simulink model "main_sim_adapt_Gref_SP"  (Simulink 7.2)
settings: Solver=ode2  SolverMode=SingleTasking  StartTime=0.0  StopTime=tsim_max  FixedStep=dtsim  RelTol=1e-3
StopFcn:
  | %mkplt
values from neighbouring files (symbols this model uses):
  aero_surf_qbar_off = get_value('aero_surf_qbar_off')    [setup_claw.m]
  aero_surf_qbar_on = get_value('aero_surf_qbar_on')    [setup_claw.m]
  assertion_time = get_value('assertion_time')    [setup_sim.m]
  att_cmd_select = get_value('att_cmd_select')    [setup_sim.m]
  att_trim_IC = orientation.att'    [setup_claw.m]
  att_type_numbers = cell2mat(struct2cell(att_type))    [setup_constants.m]
  chi_trim_IC = orientation.Vchigam(2)    [setup_claw.m]
  command_time = engage_time + 2.0    [setup_sim.m]
  compute_all_rate_cols = get_value('compute_all_rate_cols')    [setup_claw.m]
  compute_all_vel_cols = get_value('compute_all_vel_cols')    [setup_claw.m]
  da_trim_IC = tmp(1)    [setup_claw.m]
  dc_L2W_IC = orientation.dc_L2W    [setup_claw.m]
  de_trim_IC = tmp(2)    [setup_claw.m]
  dr_trim_IC = tmp(3)    [setup_claw.m]
  dtsim = get_value('dtsim')    [setup_sim.m]
  E_trim_IC = MACH_pos_IC(2)    [setup_claw.m]
  Ed_trim_IC = MACH_vel_IC(2)    [setup_claw.m]
  gain_set = gain_set_next    (= 1)    [setup_claw.m]
  gain_var_struct = rmfield(gain_var_struct,setdiff(fieldnames(gain_var_struct),{'name','size'}))    [setup_claw.m]
  gamma_trim_IC = orientation.Vchigam(3)    [setup_claw.m]
  h_trim_IC = MACH_pos_IC(3)    [setup_claw.m]
  hd_trim_IC = MACH_vel_IC(3)    [setup_claw.m]
  ideal_vel_Kb = MACH_vel_Kb(1)    [setup_sim.m]
  MACH = rmfield(MACH,'vel_throt_lrlim')    [setup_claw.m]
  MACH_att_fb = get_value('MACH_att_fb','onerror',0)    [setup_claw.m]
  MACH_att_int_IC = (1-MACH_att_Kc).*MACH_quat_IC'    [setup_ideal.m]
  MACH_att_Kb = repval(att_kbnom,MACH.att_num_cv)    [setup_claw.m]
  MACH_att_Kc = Ki2Kc(MACH_att_Ki)    [setup_ideal.m]
  MACH_att_Ki = repval(att_fi,MACH.att_num_cv)    [setup_claw.m]
  MACH_gain_mat = vertcat(MACH_gain_mat, this_gain_mat)    [setup_claw.m]
  MACH_mass_IC = obac_params.mass_IC    [setup_claw.m]
  MACH_pos_IC = x_obac_IC(MACH.NEh_idx)    [setup_claw.m]
  MACH_pos_int_IC = (1-MACH_pos_Kc).*MACH_pos_IC' + MACH_vel_IC'./MACH_pos_Kb    [setup_ideal.m]
  MACH_pos_Kb = repval(pos_kbnom,MACH.pos_num_cv)    [setup_claw.m]
  MACH_pos_Kc = Ki2Kc(MACH_pos_Ki)    [setup_ideal.m]
  MACH_pos_Ki = repval(pos_fi,MACH.pos_num_cv)    [setup_claw.m]
  MACH_pqr_Bmat_IC = Bo(MACH.pqr_idx,MACH.pqr_u_idx)    [setup_claw.m]
  MACH_pqr_IC = pqr_trim_IC    [setup_claw.m]
  MACH_pqr_int_IC = (1-MACH_pqr_Kc).*MACH_pqr_IC'    [setup_ideal.m]
  MACH_pqr_Kb = repval(pqr_kbnom,MACH.pqr_num_cv)    [setup_claw.m]
  MACH_pqr_Kc = Ki2Kc(MACH_pqr_Ki)    [setup_ideal.m]
  MACH_pqr_Ki = repval(pqr_fi,MACH.pqr_num_cv)    [setup_claw.m]
  MACH_pqr_u_IC = [ vanes_trim_IC; tvc_trim_IC; rcs_trim_IC ]    [setup_claw.m]
  MACH_quat_IC = quat_trim_IC    [setup_claw.m]
  MACH_throttle_IC = throttle_trim_IC    [setup_claw.m]
  MACH_U_nom_IC = zeros(MACH.num_u,1)    [setup_claw.m]
  MACH_vel_Bmat_IC = MACH_vel_Bmat_IC*inv(vel_perts)    [setup_claw.m]
  MACH_vel_cvdnom_IC = repval(get_value('vel_cvdnom_IC','onerror',MACH_vel_cvdnom_IC),length(MACH_vel_cvdnom_IC))'    [setup_claw.m]
  MACH_vel_IC = orientation.NdEdhd'    [setup_claw.m]
  MACH_vel_int_IC = (1-MACH_vel_Kc).*MACH_vel_IC'    [setup_ideal.m]
  MACH_vel_Kb = repval(vel_kbnom,MACH.vel_num_cv)    [setup_claw.m]
  MACH_vel_Kc = Ki2Kc(MACH_vel_Ki)    [setup_ideal.m]
  MACH_vel_Ki = repval(vel_fi,MACH.vel_num_cv)    [setup_claw.m]
  MACH_vel_uold_IC = [ MACH_quat_IC; MACH_throttle_IC ]    [setup_claw.m]
  N_trim_IC = MACH_pos_IC(1)    [setup_claw.m]
  Nd_trim_IC = MACH_vel_IC(1)    [setup_claw.m]
  obac_params = define_model('obac', get_value('obac_model_type'))    [setup_claw.m]
  pos_cmd_select = get_value('pos_cmd_select')    [setup_sim.m]
  pqr_trim_IC = [ 0 0 0 ]'    [setup_claw.m]
  rate_cmd_select = get_value('rate_cmd_select')    [setup_sim.m]
  rcs_cvddes_thresh = get_value('rcs_cvddes_thresh')    [setup_claw.m]
  reset_camcmd_on_entry = get_value('reset_camcmd_on_entry')    [setup_claw.m]
  throttle_trim_IC = u_obac_IC(MACH.throttle_idx)    [setup_claw.m]
  trac_params = define_model('trac', get_value('trac_model_type','onerror',obac_params.model_type))    [setup_sim.m]
  use_auto_att_type = get_value('use_auto_att_type','onerror',0)    [setup_claw.m]
  use_eow_as_iv = get_value('use_eow_as_iv')    [setup_claw.m]
  use_full_surf_cmd = get_value('use_full_surf_cmd')    [setup_sim.m]
  use_nav = get_value('use_nav')    [setup_claw.m]
  use_NdEdh_pos = get_value('use_NdEdh_pos')    [setup_claw.m]
  use_pos_fltpath_lim = get_value('use_pos_fltpath_lim')    [setup_claw.m]
  use_throt_estimate = get_value('use_throt_estimate')    [setup_claw.m]
  use_variable_mass = get_value('use_variable_mass')    [setup_claw.m]
  use_wind_est = get_value('use_wind_est')    [setup_claw.m]
  V_trim_IC = orientation.Vchigam(1)    [setup_claw.m]
  vel_cmd_ramp_time = get_value('vel_cmd_ramp_time')    [setup_claw.m]
  vel_cmd_select = get_value('vel_cmd_select')    [setup_sim.m]
  x_trac_IC = x_obac_IC    [setup_sim.m]
undefined symbols (not defined in the file or in its folder): accel_cmd, alpha_trim, Am, att_type, B1, bb_ellipsoid, bb_params, Bm, C, constants, cosA, DiscIntNeverNeededParam, DZkx, DZtheta, E_rwy, Ed_cmd, eow_boundary, flag_autoadapt, flag_exsig, flag_uad, full_surf_llim, full_surf_ulim, gam_cmd_descent, gam_cmd_preflare, gamdot_cmd_descent, gamdot_cmd_flare, gamdot_cmd_preflare, Gamtheta, Gamx, hd_cmd, in_error_thresh, in_exsig_vecin, in_exsig_vecout, in_reset_stoptime, in_t_exsig, in_t_timer, in_tadaptoff_forced, in_tadapton_forced, Kb, Kxhat0, Kxnom, Kxstar, max_chi_cmd, max_LOS_rate, max_vel_cmd, min_chi_cmd, min_vel_cmd, modes, N_rwy, Nd_cmd, Nrbf, P, pos, Sig, sinA, target_pos_IC, target_range_blind, target_range_detect, target_range_homing, target_vel_IC ... (+11)
libraries: simulink x44, utility_lib x36, mach_lib x24, model_lib x13, simulink_need_slupdate x8, models x8
(part 5 of 8)

== system main_sim_adapt_Gref_SP/claw_main/input processing/mode dependent stick processing/rampin vel_cmd ==
  mode : Inport  OutDataType=sfix(16)  OutScaling=2^0
  command_in : Inport  Port=2  OutDataType=sfix(16)  OutScaling=2^0
  NEh_dot : Inport  Port=3  OutDataType=sfix(16)  OutScaling=2^0
  Compare To Constant : simulink/Logic and Bit Operations/Compare To Constant  SystemSampleTime=-1  relop=<=  const=modes.att  LogicOutDataTypeMode=boolean  ZeroCross=off
  Compare To Constant1 : simulink/Logic and Bit Operations/Compare To Constant  SystemSampleTime=-1  relop===  const=modes.vel  LogicOutDataTypeMode=boolean  ZeroCross=off
  Constant : Constant  Value=MACH.dt/max(vel_cmd_ramp_time,MACH.dt)  OutDataType=sfix(16)  OutScaling=2^0
  Constant1 : Constant  OutDataType=sfix(16)  OutScaling=2^0
  Constant2 : Constant  Value=0  OutDataType=sfix(16)  OutScaling=2^0
  Logical Operator : Logic  AllPortsSameDT=off
  MinMax : MinMax  Function=max  Inputs=2  OutDataType=sfix(16)  OutScaling=2^0
  Product : Product  OutDataType=sfix(16)  OutScaling=2^0  RndMeth=Zero
  Product1 : Product  OutDataType=sfix(16)  OutScaling=2^0  RndMeth=Zero
  Sum : Sum  Inputs=-+|  OutDataType=sfix(16)  OutScaling=2^0
  Sum2 : Sum  Inputs=|++  OutDataType=sfix(16)  OutScaling=2^0
  Sum3 : Sum  Inputs=|+-  OutDataType=sfix(16)  OutScaling=2^0
  Switch : Switch  Threshold=0.5
  Switch1 : Switch  Threshold=0.5
  Unit Delay : UnitDelay  Orientation=left  SampleTime=-1
  Unit Delay1 : UnitDelay  SampleTime=-1
  Unit Delay2 : UnitDelay  Orientation=left  SampleTime=-1
  set vel cmd : Assignment  IndexOptions=Index vector (dialog)  Indices=[1 2 4]  OutputSizes=[1 1]
  vel cmd : Selector  InputPortWidth=4  IndexOptions=Index vector (dialog)  Indices=[1 2 4]  OutputSizes=1
  command_out : Outport  OutDataType=sfix(16)  OutScaling=2^0
  wires:
  Unit Delay2/1 -> Product1/2
  Logical Operator/1 -> Switch/2, Switch1/2
  Compare To Constant1/1 -> Logical Operator/2, Product1/1
  Compare To Constant/1 -> Logical Operator/1
  Unit Delay1/1 -> Compare To Constant/1
  mode/1 -> Unit Delay1/1, Compare To Constant1/1
  Unit Delay/1 -> Switch/3
  Switch/1 -> Unit Delay/1, Product/1
  NEh_dot/1 -> Sum/2
  Sum/1 -> Switch/1
  set vel cmd/1 -> command_out/1
  vel cmd/1 -> Sum2/1, Sum/1
  command_in/1 -> set vel cmd/1, vel cmd/1
  Sum2/1 -> set vel cmd/2
  Product1/1 -> Switch1/3
  Constant1/1 -> Switch1/1
  Switch1/1 -> Sum3/1
  Product/1 -> Sum2/2
  Sum3/1 -> MinMax/2
  Constant/1 -> Sum3/2
  MinMax/1 -> Product/2, Unit Delay2/1
  Constant2/1 -> MinMax/1

== system main_sim_adapt_Gref_SP/claw_main/input processing/mode dependent stick processing/set command selection switches ==
  accel_cmd_sw : Inport  OutDataType=sfix(16)  OutScaling=2^0
  CLAW_mode : Inport  Port=2  OutDataType=sfix(16)  OutScaling=2^0
  Bus Creator : BusCreator
  Constant : Constant  Value=MACH.select_cmd_array  OutDataType=sfix(16)  OutScaling=2^0
  Demux : Demux  Outputs=[4 5 4 4]
  Reshape : Reshape
  Selector : Selector  NumberOfDimensions=2  IndexMode=Zero-based  InputPortWidth=3  IndexOptions=Select all,Index vector (port)  Indices=-1,1  OutputSizes=1
  modify for accel cmd submode : Subsystem
  select_cmd : Outport  OutDataType=sfix(16)  OutScaling=2^0
  wires:
  Constant/1 -> Selector/1
  CLAW_mode/1 -> Selector/2
  Selector/1 -> Reshape/1
  Demux/1 -> Bus Creator/1  "rate"
  Demux/2 -> Bus Creator/2  "att"
  Demux/3 -> Bus Creator/3  "vel"
  Demux/4 -> Bus Creator/4  "pos"
  Reshape/1 -> Demux/1
  modify for accel cmd submode/1(select_cmd) -> select_cmd/1
  Bus Creator/1 -> modify for accel cmd submode/1(select_cmd_in)
  accel_cmd_sw/1 -> modify for accel cmd submode/2(accel_cmd_sw)

== system main_sim_adapt_Gref_SP/claw_main/input processing/mode dependent stick processing/table iv computation ==
  x_est : Inport  OutDataType=sfix(16)  OutScaling=2^0
  Bus Creator : BusCreator  Inputs=5
  Compare To Constant : simulink/Logic and Bit Operations/Compare To Constant  SystemSampleTime=-1  relop=>=  const=eow_boundary  LogicOutDataTypeMode=boolean  ZeroCross=off
  Constant : Constant  Value=2*constants.g  OutDataType=sfix(16)  OutScaling=2^0
  Constant1 : Constant  Value=sinA  OutDataType=sfix(16)  OutScaling=2^0
  Constant2 : Constant  Value=cosA  OutDataType=sfix(16)  OutScaling=2^0
  Constant3 : Constant  Value=N_rwy  OutDataType=sfix(16)  OutScaling=2^0
  Constant4 : Constant  Value=E_rwy  OutDataType=sfix(16)  OutScaling=2^0
  Dot Product : simulink/Math Operations/Dot Product  InputSameDT=on  OutDataType=sfix(16)  OutScaling=2^-10  DoSatur=off
  PreLookup Index Search : simulink_need_slupdate/PreLookup Index Search  bpData=tbl_eow  searchMode=Binary Search  cacheBpFlag=off  outputFlag=off  IndexDataType=uint32  extrapMode=Linear Extrapolation  rangeErrorMode=None
  PreLookup Index Search1 : simulink_need_slupdate/PreLookup Index Search  bpData=tbl_X  searchMode=Binary Search  cacheBpFlag=off  outputFlag=off  IndexDataType=uint32  extrapMode=Clip to Range  rangeErrorMode=None
  Product1 : Product  OutDataType=sfix(16)  OutScaling=2^0  RndMeth=Zero
  Product2 : Product  Inputs=*/  OutDataType=sfix(16)  OutScaling=2^0  RndMeth=Zero
  Product3 : Product  OutDataType=sfix(16)  OutScaling=2^0  RndMeth=Zero
  Sum1 : Sum  Inputs=|++  OutDataType=sfix(16)  OutScaling=2^0
  Sum2 : Sum  Inputs=-+|  OutDataType=sfix(16)  OutScaling=2^0
  Sum3 : Sum  Inputs=+|+  OutDataType=sfix(16)  OutScaling=2^0
  Sum4 : Sum  Inputs=|+-  OutDataType=sfix(16)  OutScaling=2^0
  get E : Selector  InputPortWidth=13  IndexOptions=Index vector (dialog)  Indices=8  OutputSizes=1
  get N : Selector  InputPortWidth=13  IndexOptions=Index vector (dialog)  Indices=7  OutputSizes=1
  get h : Selector  InputPortWidth=13  IndexOptions=Index vector (dialog)  Indices=9  OutputSizes=1
  get uvw : Selector  InputPortWidth=13  IndexOptions=Index vector (dialog)  Indices=4:6  OutputSizes=1
  table_bus : Outport  OutDataType=sfix(16)  OutScaling=2^0
  wires:
  get uvw/1 -> Dot Product/1, Dot Product/2
  get h/1 -> Sum1/1
  Constant/1 -> Product2/2
  Dot Product/1 -> Product2/1
  Product2/1 -> Sum1/2
  x_est/1 -> get h/1, get uvw/1, get N/1, get E/1
  Sum1/1 -> PreLookup Index Search/1, Compare To Constant/1, Bus Creator/2  "eow"
  PreLookup Index Search/1 -> Bus Creator/3  "eow_idx"
  get N/1 -> Sum2/2
  Sum2/1 -> Product3/1
  Product3/1 -> Sum3/1
  Constant2/1 -> Product3/2
  get E/1 -> Sum4/1
  Product1/1 -> Sum3/2
  Constant1/1 -> Product1/1
  Constant3/1 -> Sum2/1
  Constant4/1 -> Sum4/2
  Sum4/1 -> Product1/2
  Sum3/1 -> PreLookup Index Search1/1, Bus Creator/4  "X"
  Bus Creator/1 -> table_bus/1
  PreLookup Index Search1/1 -> Bus Creator/5  "X_idx"
  Compare To Constant/1 -> Bus Creator/1  "eow_large"

== system main_sim_adapt_Gref_SP/claw_main/input processing/mode dependent stick processing/use table lookup pos cmds ==
  mode : Inport  OutDataType=sfix(16)  OutScaling=2^0
  command_in : Inport  Port=2  OutDataType=sfix(16)  OutScaling=2^0
  table_bus : Inport  Port=3  OutDataType=sfix(16)  OutScaling=2^0
  Assertion : Assertion  Enabled=off  AssertionFailFcn=assertioncb  StopWhenAssertionFail=off
  Bus Selector : BusSelector  OutputSignals=eow_idx,eow_large,X_idx,X
  Compare To Constant1 : simulink/Logic and Bit Operations/Compare To Constant  SystemSampleTime=-1  relop===  const=modes.pos  LogicOutDataTypeMode=boolean  ZeroCross=off
  Constant4 : Constant  Value=use_eow_as_iv  OutDataType=sfix(16)  OutScaling=2^0
  Logical Operator : Logic  AllPortsSameDT=off
  Relational Operator : RelationalOperator  LogicOutDataTypeMode=boolean  OutDataTypeStr=boolean
  Switch1 : Switch  Threshold=0.5
  Switch2 : Switch  Threshold=0.5
  Unit Delay : UnitDelay  SampleTime=-1
  pos cmd : Selector  InputPortWidth=4  IndexOptions=Index vector (dialog)  Indices=[1 2 4]  OutputSizes=1
  set pos cmd : Assignment  IndexOptions=Index vector (dialog)  Indices=[1 2 4]  OutputSizes=[1 1]
  use E/W to get pos cmds : Subsystem
  use X to get pos cmds : Subsystem
  command_out : Outport  OutDataType=sfix(16)  OutScaling=2^0
  wires:
  Logical Operator/1 -> Switch2/2, Unit Delay/1, Relational Operator/2
  Compare To Constant1/1 -> Logical Operator/2
  Constant4/1 -> Logical Operator/1
  mode/1 -> Compare To Constant1/1
  set pos cmd/1 -> command_out/1
  pos cmd/1 -> Switch2/3
  command_in/1 -> set pos cmd/1, pos cmd/1
  Switch2/1 -> set pos cmd/2
  use E/W to get pos cmds/1(pos_cmd_eow) -> Switch1/1
  use X to get pos cmds/1(pos_cmd_X) -> Switch1/3
  Switch1/1 -> Switch2/1
  Bus Selector/2 -> Switch1/2  "<eow_large>"
  table_bus/1 -> Bus Selector/1
  Bus Selector/1 -> use E/W to get pos cmds/1(eow_idx)  "<eow_idx>"
  Bus Selector/3 -> use X to get pos cmds/1(X_idx)  "<X_idx>"
  Bus Selector/4 -> use X to get pos cmds/2(X)  "<X>"
  Unit Delay/1 -> Relational Operator/1
  Relational Operator/1 -> Assertion/1

== system main_sim_adapt_Gref_SP/claw_main/input processing/modify limits and apply to direct commands/apply surface locking ==
  u_meas : Inport  OutDataType=sfix(16)  OutScaling=2^0
  full_surf_in : Inport  Port=2  OutDataType=sfix(16)  OutScaling=2^0
  Bus Assignment : BusAssignment  AssignedSignals=full_surf_ulim,full_surf_llim
  Bus Selector : BusSelector  OutputSignals=full_surf_ulim,full_surf_cmd,full_surf_lock,full_surf_llim
  Multiport Switch : MultiPortSwitch  zeroidx=on
  Multiport Switch1 : MultiPortSwitch  zeroidx=on
  full_surf : Outport  OutDataType=sfix(16)  OutScaling=2^0
  wires:
  full_surf_in/1 -> Bus Selector/1, Bus Assignment/1
  Multiport Switch/1 -> Bus Assignment/2
  Multiport Switch1/1 -> Bus Assignment/3
  u_meas/1 -> Multiport Switch1/4, Multiport Switch/4
  Bus Assignment/1 -> full_surf/1
  Bus Selector/3 -> Multiport Switch1/1, Multiport Switch/1  "<full_surf_lock>"
  Bus Selector/1 -> Multiport Switch/2  "<full_surf_ulim>"
  Bus Selector/2 -> Multiport Switch/3, Multiport Switch1/3  "<full_surf_cmd>"
  Bus Selector/4 -> Multiport Switch1/2  "<full_surf_llim>"

== system main_sim_adapt_Gref_SP/claw_main/input processing/modify limits and apply to direct commands/throt out of fuel limits ==
  full_surf_in : Inport  OutDataType=sfix(16)  OutScaling=2^0
  Bus Assignment : BusAssignment  AssignedSignals=full_surf_ulim,full_surf_llim
  Bus Selector3 : BusSelector  OutputSignals=full_surf_ulim,full_surf_llim
  throt out of fuel limits : model_lib/throt out of fuel limits  SystemSampleTime=-1
  full_surf : Outport  OutDataType=sfix(16)  OutScaling=2^0
  wires:
  Bus Selector3/1 -> throt out of fuel limits/1  "<full_surf_ulim>"
  Bus Selector3/2 -> throt out of fuel limits/2  "<full_surf_llim>"
  full_surf_in/1 -> Bus Selector3/1, Bus Assignment/1
  Bus Assignment/1 -> full_surf/1
  throt out of fuel limits/1 -> Bus Assignment/2
  throt out of fuel limits/2 -> Bus Assignment/3

== system main_sim_adapt_Gref_SP/claw_main/input processing/select att_type/add tiebreaker for current att_type ==
  att_type_selected : Inport  OutDataType=sfix(16)  OutScaling=2^0
  priority_in : Inport  Port=2  OutDataType=sfix(16)  OutScaling=2^0
  Assignment1 : Assignment  IndexMode=Zero-based  IndexOptions=Index vector (port)  Indices=1  OutputSizes=length(att_type_numbers)+1
  Constant1 : Constant  Value=0.5  OutDataType=sfix(16)  OutScaling=2^0
  Selector : Selector  IndexMode=Zero-based  InputPortWidth=length(att_type_numbers)+1  IndexOptions=Index vector (port)  Indices=[1 3]  OutputSizes=1
  Sum1 : Sum  Inputs=|++  OutDataType=sfix(16)  OutScaling=2^0
  Unit Delay : UnitDelay  SampleTime=-1
  priority_out : Outport  OutDataType=sfix(16)  OutScaling=2^0
  wires:
  att_type_selected/1 -> Unit Delay/1
  priority_in/1 -> Selector/1, Assignment1/1
  Selector/1 -> Sum1/1
  Constant1/1 -> Sum1/2
  Sum1/1 -> Assignment1/2
  Unit Delay/1 -> Selector/2, Assignment1/3
  Assignment1/1 -> priority_out/1

== system main_sim_adapt_Gref_SP/claw_main/input processing/select att_type/compute precond vars ==
  signal_bus : Inport  OutDataType=sfix(16)  OutScaling=2^0
  scoped_bus : Inport  Port=2  OutDataType=sfix(16)  OutScaling=2^0
  -sin_b : Selector  InputPortWidth=9  IndexOptions=Index vector (dialog)  Indices=1  OutputSizes=1
  -sin_theta : Selector  InputPortWidth=9  IndexOptions=Index vector (dialog)  Indices=7  OutputSizes=1
  Bus Creator : BusCreator  Inputs=6
  Bus Selector2 : BusSelector  OutputSignals=aero_env_est.qbar,aero_env_est.vel,aero_env_est.beta,y_meas.dircos
  Bus Selector4 : BusSelector  OutputSignals=dc_L2W
  Saturation : Saturate  UpperLimit=1  LowerLimit=-1
  Saturation1 : Saturate  UpperLimit=1  LowerLimit=-1
  Trigonometric Function : Trigonometry  Operator=cos
  abs_cos_b : Fcn  Expr=sqrt(1-u(1)^2)
  abs_cos_beta : Abs
  abs_cos_gamma_rw : Abs
  abs_cos_theta : Fcn  Expr=sqrt(1-u(1)^2)
  abs_vel_rw : Abs
  cos_gamma_rw : Selector  InputPortWidth=9  IndexOptions=Index vector (dialog)  Indices=9  OutputSizes=1
  precond_vars : Outport  OutDataType=sfix(16)  OutScaling=2^0
  wires:
  Bus Selector4/1 -> cos_gamma_rw/1  "<dc_L2W>"
  Bus Selector2/1 -> Bus Creator/1  "<qbar>"
  Bus Selector2/2 -> abs_vel_rw/1  "<vel>"
  Bus Selector2/3 -> Trigonometric Function/1  "<beta>"
  Bus Selector2/4 -> -sin_theta/1, -sin_b/1  "<dircos>"
  Trigonometric Function/1 -> abs_cos_beta/1
  -sin_b/1 -> Saturation1/1
  -sin_theta/1 -> Saturation/1
  cos_gamma_rw/1 -> abs_cos_gamma_rw/1
  abs_vel_rw/1 -> Bus Creator/2  "abs_vel_rw"
  abs_cos_beta/1 -> Bus Creator/3  "abs_cos_beta"
  abs_cos_theta/1 -> Bus Creator/4  "abs_cos_theta"
  abs_cos_b/1 -> Bus Creator/5  "abs_cos_b"
  abs_cos_gamma_rw/1 -> Bus Creator/6  "abs_cos_gamma_rw"
  Saturation/1 -> abs_cos_theta/1
  Saturation1/1 -> abs_cos_b/1
  signal_bus/1 -> Bus Selector2/1
  Bus Creator/1 -> precond_vars/1
  scoped_bus/1 -> Bus Selector4/1

== system main_sim_adapt_Gref_SP/claw_main/input processing/select att_type/evaluate preconditions ==
  precond_vars : Inport  OutDataType=sfix(16)  OutScaling=2^0
  Bus Selector5 : BusSelector  OutputSignals=abs_cos_b,abs_cos_theta,abs_vel_rw,abs_cos_beta,abs_cos_gamma_rw,qbar
  Compare To Constant : simulink/Logic and Bit Operations/Compare To Constant  SystemSampleTime=-1  relop=>=  const=1  LogicOutDataTypeMode=boolean  ZeroCross=off
  Compare To Constant1 : simulink/Logic and Bit Operations/Compare To Constant  SystemSampleTime=-1  relop=>=  const=cos(pi/3)  LogicOutDataTypeMode=boolean  ZeroCross=off
  Compare To Constant2 : simulink/Logic and Bit Operations/Compare To Constant  SystemSampleTime=-1  relop=>=  const=0.1  LogicOutDataTypeMode=boolean  ZeroCross=off
  Compare To Constant3 : simulink/Logic and Bit Operations/Compare To Constant  SystemSampleTime=-1  relop=>=  const=cos(pi/3)  LogicOutDataTypeMode=boolean  ZeroCross=off
  Compare To Constant4 : simulink/Logic and Bit Operations/Compare To Constant  SystemSampleTime=-1  relop=>=  const=cos(pi/3)  LogicOutDataTypeMode=boolean  ZeroCross=off
  Compare To Constant5 : simulink/Logic and Bit Operations/Compare To Constant  SystemSampleTime=-1  relop=>=  const=1  LogicOutDataTypeMode=boolean  ZeroCross=off
  Constant : Constant  Value=boolean(0)  OutDataType=sfix(16)  OutScaling=2^0
  Logical Operator : Logic  Inputs=4  AllPortsSameDT=off  OutDataTypeMode=boolean  OutDataTypeStr=boolean
  Mux : Mux  Inputs=6
  precond_satisfied : Outport  OutDataType=sfix(16)  OutScaling=2^0
  wires:
  Compare To Constant/1 -> Logical Operator/1
  Compare To Constant1/1 -> Logical Operator/2
  Compare To Constant2/1 -> Logical Operator/3
  Compare To Constant3/1 -> Mux/3, Mux/4
  Compare To Constant4/1 -> Mux/2
  Bus Selector5/1 -> Compare To Constant4/1  "<abs_cos_b>"
  Bus Selector5/2 -> Compare To Constant3/1  "<abs_cos_theta>"
  Bus Selector5/3 -> Compare To Constant/1  "<abs_vel_rw>"
  Bus Selector5/4 -> Compare To Constant1/1  "<abs_cos_beta>"
  Bus Selector5/5 -> Compare To Constant2/1  "<abs_cos_gamma_rw>"
  Logical Operator/1 -> Mux/5, Mux/6
  Constant/1 -> Mux/1
  Compare To Constant5/1 -> Logical Operator/4
  Bus Selector5/6 -> Compare To Constant5/1  "<qbar>"
  precond_vars/1 -> Bus Selector5/1
  Mux/1 -> precond_satisfied/1

== system main_sim_adapt_Gref_SP/claw_main/input processing/select att_type/select best att_type ==
  vec : Inport  OutDataType=sfix(16)  OutScaling=2^0
  Constant4 : Constant  Value=0:length(att_type_numbers)  OutDataType=sfix(16)  OutScaling=2^0
  Constant5 : Constant  Value=length(att_type_numbers)  OutDataType=sfix(16)  OutScaling=2^0
  MinMax3 : MinMax  Function=max  OutDataType=sfix(16)  OutScaling=2^0  SaturateOnIntegerOverflow=on  InputSameDT=on
  MinMax4 : MinMax  OutDataType=sfix(16)  OutScaling=2^0  SaturateOnIntegerOverflow=on  InputSameDT=on
  Sum2 : Sum  Inputs=+-|  OutDataType=sfix(16)  OutScaling=2^0  SaturateOnIntegerOverflow=on
  argmax1 : Switch  Threshold=-eps  SaturateOnIntegerOverflow=on
  idx_max : Outport  OutDataType=sfix(16)  OutScaling=2^0
  wires:
  vec/1 -> MinMax3/1, Sum2/1
  Sum2/1 -> argmax1/2
  Constant4/1 -> argmax1/1
  Constant5/1 -> argmax1/3
  argmax1/1 -> MinMax4/1
  MinMax3/1 -> Sum2/2
  MinMax4/1 -> idx_max/1

== system main_sim_adapt_Gref_SP/claw_main/input processing/set control parameters/accel submode setup ==
  signal_bus : Inport  OutDataType=sfix(16)  OutScaling=2^0
  Bus Selector1 : BusSelector  OutputSignals=mode_sw.enable_homing_sw,mode_sw.accel_submode,mode_sw.CLAW_mode
  Constant1 : Constant  Value=3  OutDataType=sfix(16)  OutScaling=2^0
  Constant2 : Constant  Value=0  OutDataType=sfix(16)  OutScaling=2^0
  Merge1 : Merge  Inputs=3  InitialOutput=zeros(3,1)
  Merge2 : Merge  Inputs=3  InitialOutput=zeros(3,1)
  NED_dd/vchigam_dot : Subsystem  TreatAsAtomicUnit=on
  Switch : Switch  Threshold=0.5
  Switch Case : SwitchCase  CaseConditions={[1 2],3}
  Switch1 : Switch  Threshold=0.5  InputSameDT=on
  homing : Subsystem  TreatAsAtomicUnit=on
  normal vel desdyn : Subsystem  TreatAsAtomicUnit=on
  accel_cmd_sw : Outport  OutDataType=sfix(16)  OutScaling=2^0
  accel_cmd : Outport  Port=2  OutDataType=sfix(16)  OutScaling=2^0
  wires:
  Constant1/1 -> Switch/1
  Bus Selector1/1 -> Switch/2  "<enable_homing_sw>"
  Bus Selector1/2 -> Switch/3  "<accel_submode>"
  Switch/1 -> Switch1/1
  Switch1/1 -> Switch Case/1, NED_dd/vchigam_dot/1(case)
  Switch Case/1 -> NED_dd/vchigam_dot/Action
  Switch Case/2 -> homing/Action
  Switch Case/3 -> normal vel desdyn/Action
  Merge1/1 -> accel_cmd/1
  Merge2/1 -> accel_cmd_sw/1
  NED_dd/vchigam_dot/1(accel_cmd_sw) -> Merge2/1
  normal vel desdyn/2(accel_cmd) -> Merge1/3
  NED_dd/vchigam_dot/2(accel_cmd) -> Merge1/1
  homing/2(accel_cmd) -> Merge1/2
  homing/1(accel_cmd_sw) -> Merge2/2
  normal vel desdyn/1(accel_cmd_sw) -> Merge2/3
  Bus Selector1/3 -> Switch1/2  "<CLAW_mode>"
  Constant2/1 -> Switch1/3
  signal_bus/1 -> Bus Selector1/1, NED_dd/vchigam_dot/2(signal_bus), homing/1(signal_bus)

== system main_sim_adapt_Gref_SP/claw_main/input processing/set control parameters/modify MACH_att_Kf ==
  gain_bus_in : Inport  OutDataType=sfix(16)  OutScaling=2^0
  signal_bus : Inport  Port=2  OutDataType=sfix(16)  OutScaling=2^0
  Bus Assignment : BusAssignment  AssignedSignals=MACH_att_Kf
  Bus Selector : BusSelector  OutputSignals=mode_sw.att_type
  Bus Selector1 : BusSelector  OutputSignals=MACH_att_Kf
  Compare To Constant : simulink/Logic and Bit Operations/Compare To Constant  SystemSampleTime=-1  relop=>=  const=att_type.mba_bank  LogicOutDataTypeMode=boolean  ZeroCross=off
  Constant : Constant  Value=MACH_att_fb  OutDataType=sfix(16)  OutScaling=2^0
  Logical Operator : Logic  AllPortsSameDT=off
  Logical Operator1 : Logic  Operator=OR  AllPortsSameDT=off  OutDataTypeMode=boolean  OutDataTypeStr=boolean
  Logical Operator2 : Logic  Operator=NOT  AllPortsSameDT=off  OutDataTypeMode=boolean  OutDataTypeStr=boolean
  Logical Operator3 : Logic  AllPortsSameDT=off  OutDataTypeMode=boolean  OutDataTypeStr=boolean
  gain_bus : Outport  OutDataType=sfix(16)  OutScaling=2^0
  wires:
  Bus Selector1/1 -> Logical Operator/1  "<MACH_att_Kf>"
  Constant/1 -> Logical Operator2/1, Logical Operator3/1
  Logical Operator2/1 -> Logical Operator1/1
  gain_bus_in/1 -> Bus Assignment/1, Bus Selector1/1
  signal_bus/1 -> Bus Selector/1
  Bus Selector/1 -> Compare To Constant/1  "<att_type>"
  Logical Operator3/1 -> Logical Operator1/2
  Compare To Constant/1 -> Logical Operator3/2
  Logical Operator1/1 -> Logical Operator/2
  Logical Operator/1 -> Bus Assignment/2
  Bus Assignment/1 -> gain_bus/1

== system main_sim_adapt_Gref_SP/claw_main/input processing/set control parameters/select gains ==
  note: Note: Current variable gain structure will use gain_set = 1
      | if it exists, when enable_bb is true, otherwise gain_set = 0
      | (which is the global or selected default)
  enable_bb : Inport  OutDataType=sfix(16)  OutScaling=2^0
  gain_set_in : Inport  Port=2  OutDataType=sfix(16)  OutScaling=2^0
  Constant2 : Constant  Value=MACH_gain_mat  OutDataType=sfix(16)  OutScaling=2^0
  MinMax : MinMax  Inputs=2  OutDataType=sfix(16)  OutScaling=2^0
  Product : Product  Inputs=*/  OutDataType=sfix(16)  OutScaling=2^0  RndMeth=Zero
  Reshape : Reshape
  Switch : Switch
  Width1 : Width
  Width2 : Width
  mux to bus : Subsystem  mask{var_struct=gain_var_struct}
      mask prompts: var_struct "var struct"
      mask init:
      | if(~isstruct(var_struct) || length(var_struct) == 0 || ~isfield(var_struct,'name') || ~isfield(var_struct,'size'))
      |     error('var struct must be at least size 1, and must have the ''name'' and ''size'' fields defined.');
      | end
      | 
      | var_name = {var_struct.name};
      | var_size = prod(vertcat(var_struct.size),2);
      | nvar = length(var_name);
      | 
      | % remove old lines
      | nvar_old = length(get_param([gcb '/Demux'],'Outputs'));
      | for i = 1:nvar_old
      |     try
      |         delete_line(gcb,['Demux/' num2str(i)] ,['Bus Creator/' num2str(i)])
      |     end
      | end
      | 
      | set_param([gcb '/Demux'],'Outputs',mat2str(var_size));
      | set_param([gcb '/Bus Creator'],'Inputs',num2str(nvar));
      | port_handle = getfield(get_param([gcb '/Demux'],'PortHandles'),'Outport');
      | for i = 1:nvar
      |     try
      |         add_line(gcb,['Demux/' num2str(i)] ,['Bus Creator/' num2str(i)])
      |     end
      |     set(port_handle(i),'Name',var_name{i});
      | end
  select gain set : Selector  NumberOfDimensions=2  IndexMode=Zero-based  InputPortWidth=3  IndexOptions=Index vector (port),Select all  Indices=gain_set,-1  OutputSizes=1
  gain_set : Outport  OutDataType=sfix(16)  OutScaling=2^0
  gain_bus : Outport  Port=2  OutDataType=sfix(16)  OutScaling=2^0
  wires:
  Constant2/1 -> select gain set/1, Width2/1
  select gain set/1 -> Reshape/1
  Reshape/1 -> mux to bus/1(mux_in), Width1/1
  MinMax/1 -> gain_set/1, select gain set/2
  enable_bb/1 -> Switch/3
  mux to bus/1(bus_out) -> gain_bus/1
  Width2/1 -> Product/1
  Width1/1 -> Product/2
  gain_set_in/1 -> Switch/1, Switch/2
  Switch/1 -> MinMax/1
  Product/1 -> MinMax/2

== system main_sim_adapt_Gref_SP/claw_main/input processing/set control parameters/set att desdyn params ==
  gain_bus : Inport  OutDataType=sfix(16)  OutScaling=2^0
  Bus Creator : BusCreator  Inputs=7
  Bus Selector : BusSelector  OutputSignals=MACH_att_Kb,MACH_att_Ki,MACH_att_Kaw,MACH_att_Kf
  Constant1 : Constant  Value=zeros(1,4)  OutDataType=sfix(16)  OutScaling=2^0
  Constant6 : Constant  Value=MACH_quat_IC  OutDataType=sfix(16)  OutScaling=2^0
  Signal Specification : SignalSpecification  OutDataType=sfix(16)  OutScaling=2^0
  Signal Specification1 : SignalSpecification  OutDataType=sfix(16)  OutScaling=2^0
  Signal Specification2 : SignalSpecification  OutDataType=sfix(16)  OutScaling=2^0
  compute dependent gains : mach_lib/compute dependent gains  SystemSampleTime=-1
  params : Outport  OutDataType=sfix(16)  OutScaling=2^0
  wires:
  compute dependent gains/4 -> Bus Creator/6  "x0"
  Bus Selector/3 -> compute dependent gains/3  "<MACH_att_Kaw>"
  compute dependent gains/2 -> Bus Creator/4  "ki_trim"
  compute dependent gains/1 -> Bus Creator/3  "kc"
  Bus Creator/1 -> params/1
  Bus Selector/1 -> Signal Specification/1  "<MACH_att_Kb>"
  Bus Selector/2 -> Signal Specification1/1  "<MACH_att_Ki>"
  compute dependent gains/3 -> Bus Creator/5  "kaw"
  Bus Selector/4 -> Signal Specification2/1, compute dependent gains/4  "<MACH_att_Kf>"
  gain_bus/1 -> Bus Selector/1
  Signal Specification/1 -> Bus Creator/1, compute dependent gains/2  "kb"
  Signal Specification1/1 -> Bus Creator/2, compute dependent gains/1  "ki"
  Signal Specification2/1 -> Bus Creator/7  "kf"
  Constant6/1 -> compute dependent gains/5
  Constant1/1 -> compute dependent gains/6

== system main_sim_adapt_Gref_SP/claw_main/input processing/set control parameters/set pos desdyn params ==
  gain_bus : Inport  OutDataType=sfix(16)  OutScaling=2^0
  Bus Creator : BusCreator  Inputs=7
  Bus Selector : BusSelector  OutputSignals=MACH_pos_Kb,MACH_pos_Ki,MACH_pos_Kaw,MACH_pos_Kf
  Constant3 : Constant  Value=MACH_vel_IC  OutDataType=sfix(16)  OutScaling=2^0
  Constant6 : Constant  Value=MACH_pos_IC  OutDataType=sfix(16)  OutScaling=2^0
  Signal Specification : SignalSpecification  OutDataType=sfix(16)  OutScaling=2^0
  Signal Specification1 : SignalSpecification  OutDataType=sfix(16)  OutScaling=2^0
  Signal Specification2 : SignalSpecification  OutDataType=sfix(16)  OutScaling=2^0
  compute dependent gains : mach_lib/compute dependent gains  SystemSampleTime=-1
  params : Outport  OutDataType=sfix(16)  OutScaling=2^0
  wires:
  Bus Selector/3 -> compute dependent gains/3  "<MACH_pos_Kaw>"
  compute dependent gains/2 -> Bus Creator/4  "ki_trim"
  compute dependent gains/1 -> Bus Creator/3  "kc"
  Bus Creator/1 -> params/1
  Bus Selector/1 -> Signal Specification/1  "<MACH_pos_Kb>"
  Bus Selector/2 -> Signal Specification1/1  "<MACH_pos_Ki>"
  compute dependent gains/3 -> Bus Creator/5  "kaw"
  Bus Selector/4 -> Signal Specification2/1, compute dependent gains/4  "<MACH_pos_Kf>"
  compute dependent gains/4 -> Bus Creator/6  "x0"
  gain_bus/1 -> Bus Selector/1
  Signal Specification/1 -> Bus Creator/1, compute dependent gains/2  "kb"
  Signal Specification1/1 -> compute dependent gains/1, Bus Creator/2  "ki"
  Signal Specification2/1 -> Bus Creator/7  "kf"
  Constant6/1 -> compute dependent gains/5
  Constant3/1 -> compute dependent gains/6

== system main_sim_adapt_Gref_SP/claw_main/input processing/set control parameters/set rate desdyn params ==
  gain_bus : Inport  OutDataType=sfix(16)  OutScaling=2^0
  Bus Creator : BusCreator  Inputs=7
  Bus Selector : BusSelector  OutputSignals=MACH_pqr_Kb,MACH_pqr_Ki,MACH_pqr_Kaw,MACH_pqr_Kf
  Constant1 : Constant  Value=zeros(1,3)  OutDataType=sfix(16)  OutScaling=2^0
  Constant6 : Constant  Value=MACH_pqr_IC  OutDataType=sfix(16)  OutScaling=2^0
  Signal Specification : SignalSpecification  OutDataType=sfix(16)  OutScaling=2^0
  Signal Specification1 : SignalSpecification  OutDataType=sfix(16)  OutScaling=2^0
  Signal Specification2 : SignalSpecification  OutDataType=sfix(16)  OutScaling=2^0
  compute dependent gains : mach_lib/compute dependent gains  SystemSampleTime=-1
  params : Outport  OutDataType=sfix(16)  OutScaling=2^0
  wires:
  Bus Selector/4 -> Signal Specification2/1  "<MACH_pqr_Kf>"
  compute dependent gains/3 -> Bus Creator/5  "kaw"
  Signal Specification1/1 -> compute dependent gains/1, Bus Creator/2  "ki"
  Signal Specification/1 -> compute dependent gains/2, Bus Creator/1  "kb"
  Bus Creator/1 -> params/1
  compute dependent gains/1 -> Bus Creator/3  "kc"
  compute dependent gains/2 -> Bus Creator/4  "ki_trim"
  Bus Selector/3 -> compute dependent gains/3  "<MACH_pqr_Kaw>"
  compute dependent gains/4 -> Bus Creator/6  "x0"
  gain_bus/1 -> Bus Selector/1
  Bus Selector/1 -> Signal Specification/1  "<MACH_pqr_Kb>"
  Bus Selector/2 -> Signal Specification1/1  "<MACH_pqr_Ki>"
  Signal Specification2/1 -> Bus Creator/7, compute dependent gains/4  "kf"
  Constant6/1 -> compute dependent gains/5
  Constant1/1 -> compute dependent gains/6

== system main_sim_adapt_Gref_SP/claw_main/input processing/set control parameters/set rate di params ==
  full_surf : Inport  OutDataType=sfix(16)  OutScaling=2^0
  aero_env_est : Inport  Port=2  OutDataType=sfix(16)  OutScaling=2^0
  Bus Creator1 : BusCreator  Inputs=7
  Bus Selector1 : BusSelector  OutputSignals=full_surf_ulim,full_surf_llim
  Bus Selector2 : BusSelector  OutputSignals=full_surf_urlim,full_surf_lrlim
  Bus Selector3 : BusSelector  OutputSignals=qbar
  Constant5 : Constant  Value=MACH.pqr_wght_cv  OutDataType=sfix(16)  OutScaling=2^0
  Relay : Relay  OnSwitchValue=aero_surf_qbar_on  OffSwitchValue=aero_surf_qbar_off  OnOutputValue=0  OffOutputValue=1  OutDataType=sfix(16)  OutScaling=2^0
  Selector{1..2,5..6} (4 alike) : Selector  InputPortWidth=MACH.num_u  IndexOptions=Index vector (dialog)  Indices=MACH.pqr_u_idx  OutputSizes=1
  fix aero surfs when low qbar : Subsystem
  limit schedule : model_lib/no limit schedule  SystemSampleTime=-1
  select u_pref : Subsystem
  rate_params : Outport  OutDataType=sfix(16)  OutScaling=2^0
  wires:
  select u_pref/2(wght_u_pref) -> Bus Creator1/6  "wght_u_pref"
  select u_pref/1(u_pref) -> Bus Creator1/5, fix aero surfs when low qbar/4(pqr_u_pref)  "u_pref"
  Bus Creator1/1 -> rate_params/1
  full_surf/1 -> Bus Selector1/1, Bus Selector2/1, select u_pref/3(full_surf)
  Selector6/1 -> limit schedule/2
  Bus Selector1/1 -> Selector5/1  "<full_surf_ulim>"
  Bus Selector1/2 -> Selector6/1  "<full_surf_llim>"
  Selector5/1 -> limit schedule/1
  aero_env_est/1 -> select u_pref/2(aero_env_est), limit schedule/3, Bus Selector3/1
  Selector1/1 -> Bus Creator1/1  "u_urlim"
  Selector2/1 -> Bus Creator1/2  "u_lrlim"
  fix aero surfs when low qbar/1(pqr_u_ulim) -> Bus Creator1/3  "u_ulim"
  fix aero surfs when low qbar/2(pqr_u_llim) -> Bus Creator1/4  "u_llim"
  limit schedule/1 -> fix aero surfs when low qbar/1(pqr_u_ulim_in)
  limit schedule/2 -> fix aero surfs when low qbar/2(pqr_u_llim_in)
  Bus Selector2/1 -> Selector1/1  "<full_surf_urlim>"
  Bus Selector2/2 -> Selector2/1  "<full_surf_lrlim>"
  Constant5/1 -> Bus Creator1/7  "wght_cv"
  Bus Selector3/1 -> Relay/1  "<qbar>"
  Relay/1 -> fix aero surfs when low qbar/3(low_qbar), select u_pref/1(low_qbar)

== system main_sim_adapt_Gref_SP/claw_main/input processing/set control parameters/set vel desdyn params ==
  gain_bus : Inport  OutDataType=sfix(16)  OutScaling=2^0
  Bus Creator : BusCreator  Inputs=7
  Bus Selector : BusSelector  OutputSignals=MACH_vel_Kb,MACH_vel_Ki,MACH_vel_Kaw,MACH_vel_Kf
  Constant1 : Constant  Value=MACH_vel_cvdnom_IC  OutDataType=sfix(16)  OutScaling=2^0
  Constant6 : Constant  Value=MACH_vel_IC  OutDataType=sfix(16)  OutScaling=2^0
  Signal Specification : SignalSpecification  OutDataType=sfix(16)  OutScaling=2^0
  Signal Specification1 : SignalSpecification  OutDataType=sfix(16)  OutScaling=2^0
  Signal Specification2 : SignalSpecification  OutDataType=sfix(16)  OutScaling=2^0
  compute dependent gains : mach_lib/compute dependent gains  SystemSampleTime=-1
  params : Outport  OutDataType=sfix(16)  OutScaling=2^0
  wires:
  Bus Selector/4 -> Signal Specification2/1, compute dependent gains/4  "<MACH_vel_Kf>"
  compute dependent gains/3 -> Bus Creator/5  "kaw"
  Bus Selector/2 -> Signal Specification1/1  "<MACH_vel_Ki>"
  Bus Selector/1 -> Signal Specification/1  "<MACH_vel_Kb>"
  Bus Creator/1 -> params/1
  compute dependent gains/1 -> Bus Creator/3  "kc"
  compute dependent gains/2 -> Bus Creator/4  "ki_trim"
  Bus Selector/3 -> compute dependent gains/3  "<MACH_vel_Kaw>"
  gain_bus/1 -> Bus Selector/1
  Signal Specification/1 -> Bus Creator/1, compute dependent gains/2  "kb"
  Signal Specification1/1 -> compute dependent gains/1, Bus Creator/2  "ki"
  Signal Specification2/1 -> Bus Creator/7  "kf"
  compute dependent gains/4 -> Bus Creator/6  "x0"
  Constant6/1 -> compute dependent gains/5
  Constant1/1 -> compute dependent gains/6

== system main_sim_adapt_Gref_SP/claw_main/rate_loops/B matrix comp/cvd_def_nom ==
  x : Inport  OutDataType=sfix(16)  OutScaling=2^0
  u : Inport  Port=2  OutDataType=sfix(16)  OutScaling=2^0
  xdot : Inport  Port=3  OutDataType=sfix(16)  OutScaling=2^0
  Selector : Selector  InputPortWidth=MACH.num_x  IndexOptions=Index vector (dialog)  Indices=MACH.pqr_idx  OutputSizes=1
  Terminator : Terminator
  Terminator1 : Terminator
  cvd : Outport  OutDataType=sfix(16)  OutScaling=2^0
  wires:
  xdot/1 -> Selector/1
  Selector/1 -> cvd/1
  u/1 -> Terminator/1
  x/1 -> Terminator1/1

== system main_sim_adapt_Gref_SP/claw_main/rate_loops/B matrix comp/cvd_def_pert ==
  x : Inport  OutDataType=sfix(16)  OutScaling=2^0
  u : Inport  Port=2  OutDataType=sfix(16)  OutScaling=2^0
  xdot : Inport  Port=3  OutDataType=sfix(16)  OutScaling=2^0
  Selector : Selector  InputPortWidth=MACH.num_x  IndexOptions=Index vector (dialog)  Indices=MACH.pqr_idx  OutputSizes=1
  Terminator : Terminator
  Terminator1 : Terminator
  cvd : Outport  OutDataType=sfix(16)  OutScaling=2^0
  wires:
  xdot/1 -> Selector/1
  Selector/1 -> cvd/1
  u/1 -> Terminator/1
  x/1 -> Terminator1/1

== system main_sim_adapt_Gref_SP/claw_main/rate_loops/B matrix comp/pert insert ==
  X_nom : Inport  OutDataType=sfix(16)  OutScaling=2^0
  U_nom : Inport  Port=2  OutDataType=sfix(16)  OutScaling=2^0
  D_pert : Inport  Port=3  OutDataType=sfix(16)  OutScaling=2^0
  Assignment : Assignment  IndexOptions=Index vector (dialog)  Indices=MACH.pqr_u_idx  OutputSizes=[1 1]
  X_pert : Outport  OutDataType=sfix(16)  OutScaling=2^0
  U_pert : Outport  Port=2  OutDataType=sfix(16)  OutScaling=2^0
  wires:
  D_pert/1 -> Assignment/2
  Assignment/1 -> U_pert/1
  X_nom/1 -> X_pert/1
  U_nom/1 -> Assignment/1

== system main_sim_adapt_Gref_SP/claw_main/rate_loops/B matrix comp/pert_comp ==
  col : Inport  OutDataType=sfix(16)  OutScaling=2^0
  d_nom : Inport  Port=2  OutDataType=sfix(16)  OutScaling=2^0
  params : Inport  Port=3  OutDataType=sfix(16)  OutScaling=2^0
  Bus Selector : BusSelector  OutputSignals=u_ulim,u_llim
  Constant2 : Constant  Value=diag(MACH.pqr_u_pert)  OutDataType=sfix(16)  OutScaling=2^0
  pick +/- pert : mach_lib/pick +//- pert  SystemSampleTime=-1  num_u=MACH.pqr_num_u
  d_pert : Outport  OutDataType=sfix(16)  OutScaling=2^0
  d_div : Outport  Port=2  OutDataType=sfix(16)  OutScaling=2^0
  wires:
  Constant2/1 -> pick +/- pert/5
  pick +/- pert/1 -> d_pert/1
  pick +/- pert/2 -> d_div/1  "scalar pert value"
  col/1 -> pick +/- pert/1
  d_nom/1 -> pick +/- pert/2
  Bus Selector/1 -> pick +/- pert/3  "<u_ulim>"
  params/1 -> Bus Selector/1
  Bus Selector/2 -> pick +/- pert/4  "<u_llim>"

== system main_sim_adapt_Gref_SP/claw_main/rate_loops/P+I+AW+TRIM Control/variable gain comp ==
  int : Inport  OutDataType=sfix(16)  OutScaling=2^0
  cv : Inport  Port=2  OutDataType=sfix(16)  OutScaling=2^0
  cvc : Inport  Port=3  OutDataType=sfix(16)  OutScaling=2^0
  kc : Inport  Port=4  OutDataType=sfix(16)  OutScaling=2^0
  kb : Inport  Port=5  OutDataType=sfix(16)  OutScaling=2^0
  ki : Inport  Port=6  OutDataType=sfix(16)  OutScaling=2^0
  Compare To Zero : simulink/Logic and Bit Operations/Compare To Zero  SystemSampleTime=-1  relop=>  LogicOutDataTypeMode=boolean  ZeroCross=off
  Compare To Zero1 : simulink/Logic and Bit Operations/Compare To Zero  SystemSampleTime=-1  relop===  LogicOutDataTypeMode=boolean  ZeroCross=off
  Demux : Demux  Outputs=2
  Gain : Gain  Gain=1/MACH.dt  ParameterDataType=sfix(16)  ParameterScaling=2^0  OutDataType=sfix(16)  OutScaling=2^0
  Mux : Mux  Inputs=2
  Mux1 : Mux  Inputs=2
  Product1 : Product  Inputs=*/  OutDataType=sfix(16)  OutScaling=2^0  RndMeth=Zero
  Product2 : Product  Inputs=3  OutDataType=sfix(16)  OutScaling=2^0  RndMeth=Zero
  Product3 : Product  Inputs=3  OutDataType=sfix(16)  OutScaling=2^0  RndMeth=Zero
  Product5 : Product  OutDataType=sfix(16)  OutScaling=2^0  RndMeth=Zero
  Sum : Sum  Inputs=|++  OutDataType=sfix(16)  OutScaling=2^0
  Sum1 : Sum  Inputs=|+-  OutDataType=sfix(16)  OutScaling=2^0
  Sum2 : Sum  Inputs=|-+  OutDataType=sfix(16)  OutScaling=2^0
  Sum6 : Sum  Inputs=-+|  OutDataType=sfix(16)  OutScaling=2^0
  Unit Delay : UnitDelay  SampleTime=-1
  int_incr : Outport  OutDataType=sfix(16)  OutScaling=2^0
  wires:
  Gain/1 -> Sum1/1
  Product1/1 -> Gain/1
  Product3/1 -> Sum1/2
  Compare To Zero1/1 -> Product3/3
  ki/1 -> Compare To Zero1/1
  Sum1/1 -> int_incr/1
  Demux/2 -> Sum/2
  Demux/1 -> Sum/1
  Product2/1 -> Demux/1
  Mux1/1 -> Product2/1
  Unit Delay/1 -> Sum6/2, Compare To Zero/1
  Sum6/1 -> Product2/2
  Product5/1 -> Mux/1
  kc/1 -> Product5/1
  kb/1 -> Product5/2, Product3/1, Mux/2, Product1/2
  Sum/1 -> Product1/1
  Compare To Zero/1 -> Product2/3
  cv/1 -> Sum2/1
  Sum2/1 -> Mux1/2
  int/1 -> Product3/2, Sum2/2
  Mux/1 -> Unit Delay/1, Sum6/1
  cvc/1 -> Mux1/1

== system main_sim_adapt_Gref_SP/claw_main/rate_loops/allocation/RCS allocation ==
  Bmat : Inport  OutDataType=sfix(16)  OutScaling=2^0
  rcs_cmd_old : Inport  Port=2  OutDataType=sfix(16)  OutScaling=2^0
  cvd_des : Inport  Port=3  OutDataType=sfix(16)  OutScaling=2^0
  params : Inport  Port=4  OutDataType=sfix(16)  OutScaling=2^0
  Bus Selector : BusSelector  OutputSignals=wght_cv,u_ulim,u_llim
  Constant : Constant  Value=[1 1 1]  OutDataType=sfix(16)  OutScaling=2^0
  Constant1 : Constant  Value=MACH.pqr_rcs_use  OutDataType=sfix(16)  OutScaling=2^0
  Constant2 : Constant  Value=rcs_cvddes_thresh  OutDataType=sfix(16)  OutScaling=2^0
  Embedded MATLAB Function : Stateflow chart
  Sum5 : Sum  Inputs=+-|  OutDataType=sfix(16)  OutScaling=2^0  SaturateOnIntegerOverflow=on  InputSameDT=on  OutDataTypeStr=Inherit: Same as first input
  Terminator{,1..3} (4 alike) : Terminator
  rcs_cmd : Outport  OutDataType=sfix(16)  OutScaling=2^0
  cvd_extra : Outport  Port=2  OutDataType=sfix(16)  OutScaling=2^0
  wires:
  Embedded MATLAB Function/3(scale) -> Terminator3/1
  params/1 -> Bus Selector/1
  cvd_des/1 -> Sum5/2, Embedded MATLAB Function/5(cvd_des)
  Sum5/1 -> cvd_extra/1
  Bmat/1 -> Embedded MATLAB Function/1(Bmat)
  Embedded MATLAB Function/1(rcs_cmd) -> rcs_cmd/1
  Embedded MATLAB Function/2(minerr) -> Terminator2/1
  Embedded MATLAB Function/4(cvd_actual) -> Sum5/1
  rcs_cmd_old/1 -> Terminator/1
  Constant2/1 -> Embedded MATLAB Function/6(err_thresh)
  Bus Selector/3 -> Embedded MATLAB Function/4(llim)  "<u_llim>"
  Bus Selector/2 -> Embedded MATLAB Function/3(ulim)  "<u_ulim>"
  Constant1/1 -> Embedded MATLAB Function/7(rcs_use_in)
  Bus Selector/1 -> Terminator1/1  "<wght_cv>"
  Constant/1 -> Embedded MATLAB Function/2(wght_cv)

== system main_sim_adapt_Gref_SP/claw_main/rate_loops/allocation/config_di ==
  cvd_nom : Inport  OutDataType=sfix(16)  OutScaling=2^0
  Bmat : Inport  Port=2  OutDataType=sfix(16)  OutScaling=2^0
  d_old : Inport  Port=3  OutDataType=sfix(16)  OutScaling=2^0
  d_nom : Inport  Port=4  OutDataType=sfix(16)  OutScaling=2^0
  cvd_des : Inport  Port=5  OutDataType=sfix(16)  OutScaling=2^0
  params : Inport  Port=6  OutDataType=sfix(16)  OutScaling=2^0
  di_smn : mach_lib/di_smn  SystemSampleTime=-1
  d_cmd : Outport  OutDataType=sfix(16)  OutScaling=2^0
  cvd_extra : Outport  Port=2  OutDataType=sfix(16)  OutScaling=2^0
  lambda : Outport  Port=3  OutDataType=sfix(16)  OutScaling=2^0
  solve_dat : Outport  Port=4  OutDataType=sfix(16)  OutScaling=2^0
  wires:
  cvd_nom/1 -> di_smn/1
  Bmat/1 -> di_smn/2
  d_old/1 -> di_smn/3
  d_nom/1 -> di_smn/4
  cvd_des/1 -> di_smn/5
  params/1 -> di_smn/6
  di_smn/1 -> d_cmd/1
  di_smn/2 -> cvd_extra/1
  di_smn/3 -> lambda/1
  di_smn/4 -> solve_dat/1

== system main_sim_adapt_Gref_SP/claw_main/rate_loops/allocation/param select rcs ==
  params_all : Inport  OutDataType=sfix(16)  OutScaling=2^0
  Bus Creator1 : BusCreator  Inputs=7
  Bus Selector : BusSelector  OutputSignals=u_ulim,u_llim,u_urlim,u_lrlim,u_pref,wght_u_pref,wght_cv
  Selector{,1..5} (6 alike) : Selector  InputPortWidth=MACH.pqr_num_u  IndexOptions=Index vector (dialog)  Indices=idx  OutputSizes=1
  params : Outport  OutDataType=sfix(16)  OutScaling=2^0
  wires:
  Bus Creator1/1 -> params/1
  Bus Selector/6 -> Selector5/1  "<wght_u_pref>"
  Bus Selector/5 -> Selector4/1  "<u_pref>"
  Bus Selector/4 -> Selector3/1  "<u_lrlim>"
  Bus Selector/3 -> Selector2/1  "<u_urlim>"
  Bus Selector/2 -> Selector1/1  "<u_llim>"
  Bus Selector/1 -> Selector/1  "<u_ulim>"
  params_all/1 -> Bus Selector/1
  Selector3/1 -> Bus Creator1/4  "u_lrlim"
  Selector2/1 -> Bus Creator1/3  "u_urlim"
  Selector/1 -> Bus Creator1/1  "u_ulim"
  Selector1/1 -> Bus Creator1/2  "u_llim"
  Selector4/1 -> Bus Creator1/5  "u_pref"
  Selector5/1 -> Bus Creator1/6  "wght_u_pref"
  Bus Selector/7 -> Bus Creator1/7  "<wght_cv>"

== system main_sim_adapt_Gref_SP/claw_main/rate_loops/allocation/param select smn ==
  params_all : Inport  OutDataType=sfix(16)  OutScaling=2^0
  Bus Creator1 : BusCreator  Inputs=7
  Bus Selector : BusSelector  OutputSignals=u_ulim,u_llim,u_urlim,u_lrlim,u_pref,wght_u_pref,wght_cv
  Selector{,1..5} (6 alike) : Selector  InputPortWidth=MACH.pqr_num_u  IndexOptions=Index vector (dialog)  Indices=idx  OutputSizes=1
  params : Outport  OutDataType=sfix(16)  OutScaling=2^0
  wires:
  Bus Selector/7 -> Bus Creator1/7  "<wght_cv>"
  Selector5/1 -> Bus Creator1/6  "wght_u_pref"
  Selector4/1 -> Bus Creator1/5  "u_pref"
  Selector1/1 -> Bus Creator1/2  "u_llim"
  Selector/1 -> Bus Creator1/1  "u_ulim"
  Selector2/1 -> Bus Creator1/3  "u_urlim"
  Selector3/1 -> Bus Creator1/4  "u_lrlim"
  params_all/1 -> Bus Selector/1
  Bus Selector/1 -> Selector/1  "<u_ulim>"
  Bus Selector/2 -> Selector1/1  "<u_llim>"
  Bus Selector/3 -> Selector2/1  "<u_urlim>"
  Bus Selector/4 -> Selector3/1  "<u_lrlim>"
  Bus Selector/5 -> Selector4/1  "<u_pref>"
  Bus Selector/6 -> Selector5/1  "<wght_u_pref>"
  Bus Creator1/1 -> params/1

== system main_sim_adapt_Gref_SP/claw_main/rate_loops/select rate cmd/get direct cmd ==
  signal_bus : Inport  OutDataType=sfix(16)  OutScaling=2^0
  Bus Selector1 : BusSelector  OutputSignals=cmd_bus.autopilot_cmd,mode_sw.full_surf_cmd_sw,full_surf.full_surf_cmd
  Demux2 : Demux  Outputs=[ 3 1 ]
  Gain1 : Gain  Gain=MACH.throt_mixer  ParameterDataType=sfix(16)  ParameterScaling=2^0  OutDataType=sfix(16)  OutScaling=2^0
  Multiport Switch2 : MultiPortSwitch  Inputs=2  zeroidx=on
  Mux2 : Mux  Inputs=2
  throttle : Selector  InputPortWidth=MACH.num_u  IndexOptions=Index vector (dialog)  Indices=MACH.throttle_idx  OutputSizes=1
  direct_cmd : Outport  OutDataType=sfix(16)  OutScaling=2^0
  wires:
  Demux2/1 -> Mux2/1
  Demux2/2 -> Gain1/1
  Mux2/1 -> direct_cmd/1
  signal_bus/1 -> Bus Selector1/1
  Bus Selector1/1 -> Demux2/1  "<autopilot_cmd>"
  Bus Selector1/2 -> Multiport Switch2/1  "<full_surf_cmd_sw>"
  Gain1/1 -> Multiport Switch2/2
  Bus Selector1/3 -> throttle/1  "<full_surf_cmd>"
  throttle/1 -> Multiport Switch2/3
  Multiport Switch2/1 -> Mux2/2

== system main_sim_adapt_Gref_SP/claw_main/state est/process sensors/compute dc_fltpath ==
  NEh_dot_fltpath : Inport  OutDataType=sfix(16)  OutScaling=2^0
  Gain : Gain  Gain=repmat([1 1 -1],3,1)  ParameterDataType=sfix(16)  ParameterScaling=2^0  OutDataType=sfix(16)  OutScaling=2^0
  Gain1 : Gain  Gain=[1 1 -1]  ParameterDataType=sfix(16)  ParameterScaling=2^0  OutDataType=sfix(16)  OutScaling=2^0
  Reshape : Reshape  OutputDimensionality=Customize  OutputDimensions=[3 3]
  Terminator : Terminator
  vec2dc : utility_lib/vec2dc  SystemSampleTime=-1
  dc_fltpath : Outport  OutDataType=sfix(16)  OutScaling=2^0
  wires:
  vec2dc/1 -> Reshape/1
  Reshape/1 -> Gain/1
  Gain1/1 -> vec2dc/1
  vec2dc/2 -> Terminator/1
  Gain/1 -> dc_fltpath/1
  NEh_dot_fltpath/1 -> Gain1/1
